simulink model "enable_test3"  (R2017b)
settings: Solver=FixedStepDiscrete  StartTime=0.0  StopTime=10.0  FixedStep=0.200000  RelTol=1e-3  EnableMultiTasking=on
settings Model: Creator=hamza  LastModifiedBy=hbourbou
settings DataIOCC: SaveFormat=StructureWithTime
settings OptimizationCC: LifeSpan=inf
settings DebuggingCC: SFUnexpectedBacktrackingDiag=warning  SFNoUnconditionalDefaultTransitionDiag=warning  SFExecutionAtInitializationDiag=none
settings HardwareCC: ProdBitPerSizeT=32  ProdBitPerPtrDiffT=32  ProdWordSize=32  ProdHWDeviceType=Specified
settings CodeAppCC: StateflowObjectComments=on
settings GRTTargetCC: TargetLangStandard=C89/C90 (ANSI)  GeneratePreprocessorConditionals=Disable all
settings ConfigComp: CovMetricSettings=dw  CovHtmlReporting=on  CovSaveCumulativeToWorkspaceVar=on  CovSaveSingleToWorkspaceVar=on  CovExternalEMLEnable=off

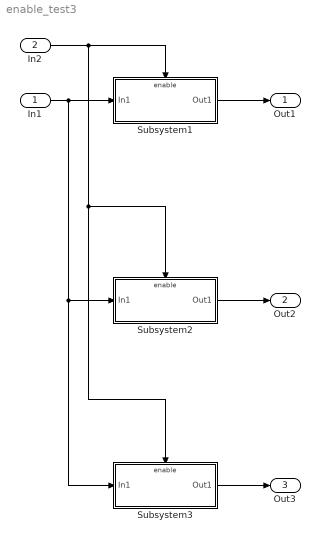
== system enable_test3 ==
  In1 : Inport  OutDataTypeStr=double
  In2 : Inport  Port=2  OutDataTypeStr=boolean
  Subsystem1 : Subsystem  TreatAsAtomicUnit=on
  Subsystem2 : Subsystem  TreatAsAtomicUnit=on
  Subsystem3 : Subsystem  TreatAsAtomicUnit=on
  Out1 : Outport
  Out2 : Outport  Port=2
  Out3 : Outport  Port=3
  wires:
  In1/1 -> Subsystem3/1(In1), Subsystem2/1(In1), Subsystem1/1(In1)
  Subsystem1/1(Out1) -> Out1/1
  Subsystem2/1(Out1) -> Out2/1
  Subsystem3/1(Out1) -> Out3/1
  In2/1 -> Subsystem3/Enable, Subsystem2/Enable, Subsystem1/Enable

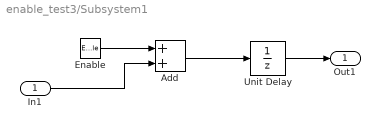
== system enable_test3/Subsystem1 ==
  In1 : Inport
  Enable : EnablePort  StatesWhenEnabling=reset  ShowOutputPort=on
  Add : Sum
  Unit Delay : UnitDelay  SampleTime=-1
  Out1 : Outport
  wires:
  Enable/1 -> Add/1
  In1/1 -> Add/2
  Add/1 -> Unit Delay/1
  Unit Delay/1 -> Out1/1

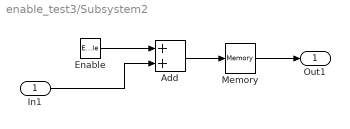
== system enable_test3/Subsystem2 ==
  In1 : Inport
  Enable : EnablePort  StatesWhenEnabling=reset  ShowOutputPort=on
  Add : Sum
  Memory : Memory
  Out1 : Outport
  wires:
  Enable/1 -> Add/1
  In1/1 -> Add/2
  Add/1 -> Memory/1
  Memory/1 -> Out1/1

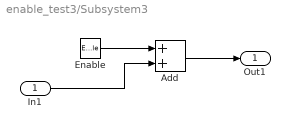
== system enable_test3/Subsystem3 ==
  In1 : Inport
  Enable : EnablePort  ShowOutputPort=on
  Add : Sum
  Out1 : Outport
  wires:
  Enable/1 -> Add/1
  In1/1 -> Add/2
  Add/1 -> Out1/1
